simulink model "model_1"  (R2020a)
settings: Solver=VariableStepAuto  StartTime=0.0  StopTime=10.0  RelTol=1e-3
settings Model: Creator=Notnik_kg  LastModifiedBy=Notnik_kg

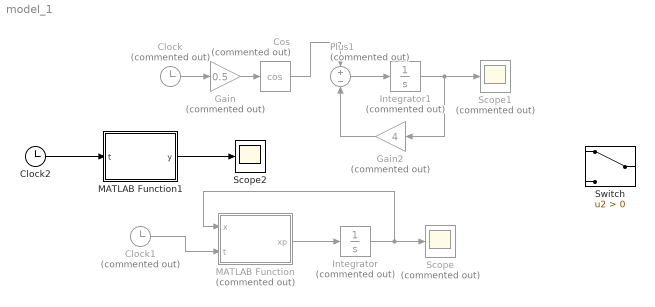
== system model_1 ==
  Clock : Clock  Commented=on
  Clock1 : Clock  Commented=on
  Clock2 : Clock
  Cos : Trigonometry  Commented=on  Operator=cos
  Gain : Gain  Commented=on  Gain=0.5
  Gain2 : Gain  Commented=on  Gain=4
  Integrator : Integrator  Commented=on  InitialCondition=1
  Integrator1 : Integrator  Commented=on  InitialCondition=1
  MATLAB Function : MATLAB Function  Commented=on  TreatAsAtomicUnit=on
  MATLAB Function1 : MATLAB Function  TreatAsAtomicUnit=on
  Plus1 : Sum  Commented=on  Inputs=+-
  Scope : Scope  Commented=on
  Scope1 : Scope  Commented=on
  Scope2 : Scope
  Switch : Switch  Criteria=u2 > Threshold
  wires:
  Integrator1/1 -> Scope1/1, Gain2/1
  Gain2/1 -> Plus1/2
  Plus1/1 -> Integrator1/1
  Clock/1 -> Gain/1
  Gain/1 -> Cos/1
  Cos/1 -> Plus1/1
  Clock1/1 -> MATLAB Function/2(t)
  MATLAB Function/1(xp) -> Integrator/1
  Integrator/1 -> Scope/1, MATLAB Function/1(x)
  Clock2/1 -> MATLAB Function1/1(t)
  MATLAB Function1/1(y) -> Scope2/1

== matlab function model_1/MATLAB Function ==
  data: x input; xp output; t input
function xp = fcn(x, t)
xp = cos(0.5.*t) - 4.*x;

== matlab function model_1/MATLAB Function1 ==
  data: t input; y output
function y = fcn(t)
y = (2.*(sin(t./2) + 8.*cos(t./2)))./65 + exp(-4.*t).*(49./65);
